simulink model "Ej3"  (R2023a)
settings: Solver=VariableStepAuto  StartTime=0.0  StopTime=20  RelTol=1e-3
settings Model: Creator=santi  LastModifiedBy=santi

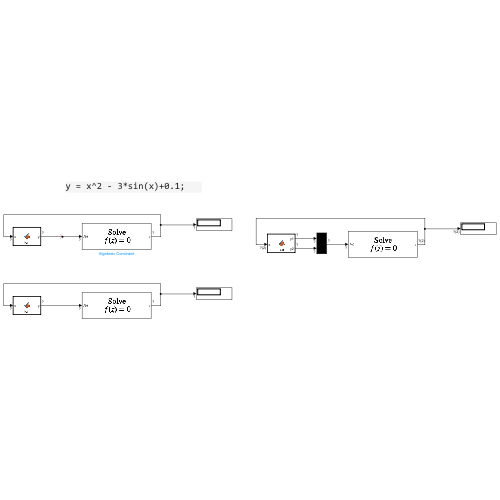
[thumbnail: Simulink's stored preview of the top-level diagram]
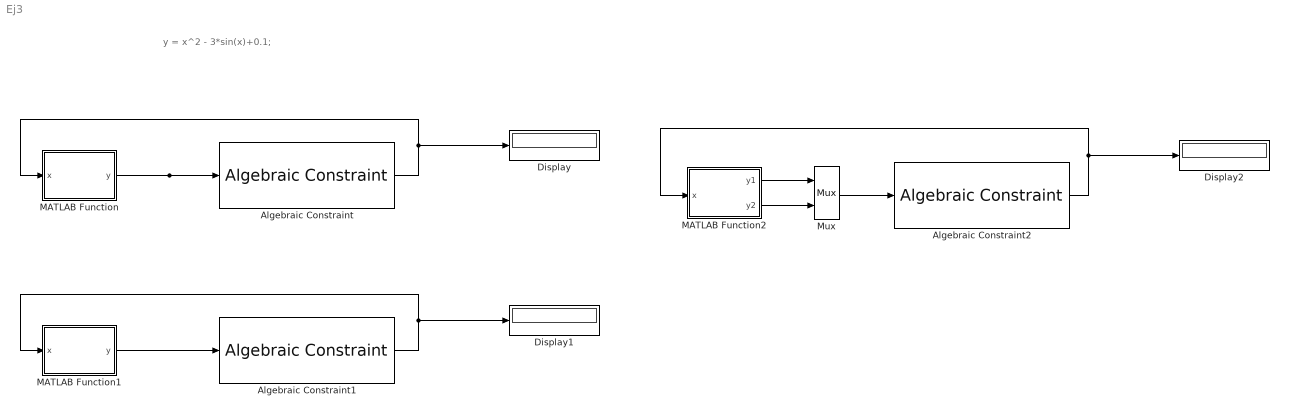
== system Ej3 ==
  note: y = x^2 - 3*sin(x)+0.1;
  Algebraic Constraint : AlgebraicConstraint  InitialGuess=-0.2
  Algebraic Constraint1 : AlgebraicConstraint  InitialGuess=1.5
  Algebraic Constraint2 : AlgebraicConstraint  InitialGuess=[-0.2 1.5]
  Display : Display
  Display1 : Display
  Display2 : Display
  MATLAB Function : MATLAB Function  TreatAsAtomicUnit=on
  MATLAB Function1 : MATLAB Function  TreatAsAtomicUnit=on
  MATLAB Function2 : MATLAB Function  TreatAsAtomicUnit=on
  Mux : Mux  Inputs=2
  wires:
  MATLAB Function/1(y) -> Algebraic Constraint/1
  Algebraic Constraint/1 -> MATLAB Function/1(x), Display/1
  Algebraic Constraint1/1 -> Display1/1, MATLAB Function1/1(x)
  MATLAB Function1/1(y) -> Algebraic Constraint1/1
  Algebraic Constraint2/1 -> Display2/1, MATLAB Function2/1(x)
  MATLAB Function2/1(y1) -> Mux/1
  MATLAB Function2/2(y2) -> Mux/2
  Mux/1 -> Algebraic Constraint2/1

== matlab function Ej3/MATLAB Function ==
  data: x input; y output
function y = fcn(x)

y = x^2 - 3*sin(x)+0.1;

== matlab function Ej3/MATLAB Function2 ==
  data: x input; y1 output; y2 output
function [y1,y2] = fcn(x)

[y1 ; y2] = x.^2 -3.*sin(x) +0.1;

== matlab function Ej3/MATLAB Function1 ==
  data: x input; y output
function y = fcn(x)

y = x^2 - 3*sin(x)+0.1;
